simulink library "btb"  (Simulink 8.1)
settings: Solver=ode1  StartTime=0.0  StopTime=Inf  FixedStep=0.001  RelTol=1e-3
PostLoadFcn:
  | , if any(exist('dsrtsu_mdlpostloadfcn', 'file') == [2, 3, 6]), try dsrtsu_mdlpostloadfcn('Execute', bdroot); catch fprintf('Error in PostLoadFcn (dsrtsu_mdlpostloadfcn) for model "%s":\n %s\n', bdroot, lasterr); end, end,
undefined symbols (not defined in the file or in its folder): KACC_ACCDefBrakDist_m, KACC_ACCStopDistance_m, KACC_BrakeToStopConsideredDecel_mps2, KACC_BrakeToStopFreeRunTime_s
libraries: hcu_lib x2
settings Model: DSRTSU_INTERNAL_RTI_VER=450  DSRTSU_INTERNAL_RTI_TYPE=rti1401  Creator=AT015555  LastModifiedBy=AT015555

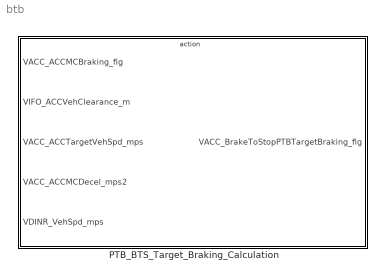
== system btb ==
  PTB_BTS_Target_Braking_Calculation : Subsystem  TreatAsAtomicUnit=on

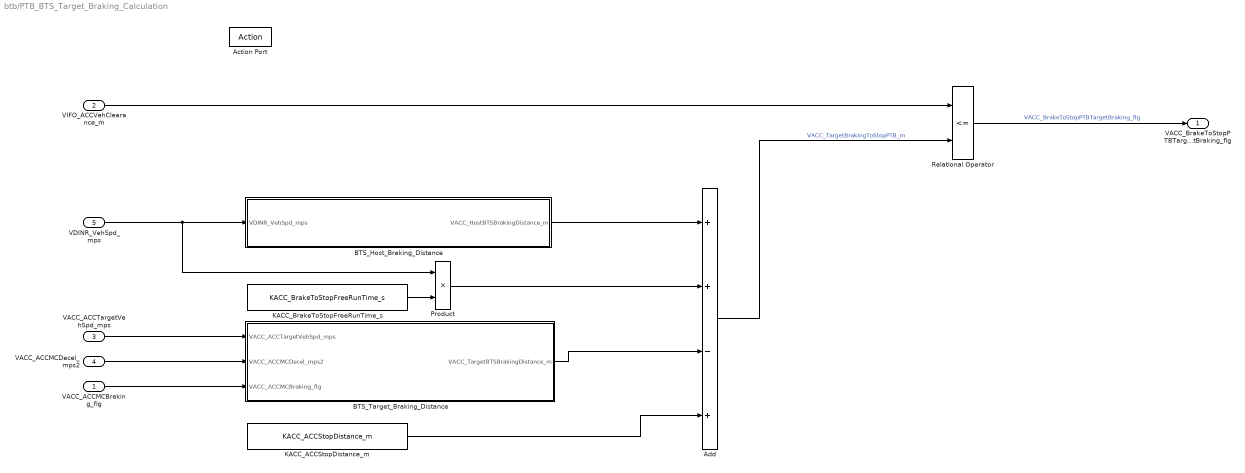
== system btb/PTB_BTS_Target_Braking_Calculation ==
  VACC_ACCMCBraking_flg : Inport
  VIFO_ACCVehClearance_m : Inport  Port=2
  VACC_ACCTargetVehSpd_mps : Inport  Port=3
  VACC_ACCMCDecel_mps2 : Inport  Port=4
  VDINR_VehSpd_mps : Inport  Port=5
  Action Port : ActionPort
  Add : Sum  Inputs=++-+
  BTS_Host_Braking_Distance : Subsystem
  BTS_Target_Braking_Distance : Subsystem
  KACC_ACCStopDistance_m : Constant  Value=KACC_ACCStopDistance_m
  KACC_BrakeToStopFreeRunTime_s : Constant  Value=KACC_BrakeToStopFreeRunTime_s
  Product : Product
  Relational Operator : RelationalOperator  Operator=<=  OutDataTypeStr=boolean
  VACC_BrakeToStopPTBTargetBraking_flg : Outport
  wires:
  VACC_ACCMCBraking_flg/1 -> BTS_Target_Braking_Distance/3(VACC_ACCMCBraking_flg)
  Relational Operator/1 -> VACC_BrakeToStopPTBTargetBraking_flg/1  "VACC_BrakeToStopPTBTargetBraking_flg"
  Add/1 -> Relational Operator/2  "VACC_TargetBrakingToStopPTB_m"
  VACC_ACCMCDecel_mps2/1 -> BTS_Target_Braking_Distance/2(VACC_ACCMCDecel_mps2)
  VACC_ACCTargetVehSpd_mps/1 -> BTS_Target_Braking_Distance/1(VACC_ACCTargetVehSpd_mps)
  BTS_Target_Braking_Distance/1(VACC_TargetBTSBrakingDistance_m) -> Add/3
  Product/1 -> Add/2
  KACC_BrakeToStopFreeRunTime_s/1 -> Product/2
  BTS_Host_Braking_Distance/1(VACC_HostBTSBrakingDistance_m) -> Add/1
  VDINR_VehSpd_mps/1 -> BTS_Host_Braking_Distance/1(VDINR_VehSpd_mps), Product/1
  KACC_ACCStopDistance_m/1 -> Add/4
  VIFO_ACCVehClearance_m/1 -> Relational Operator/1

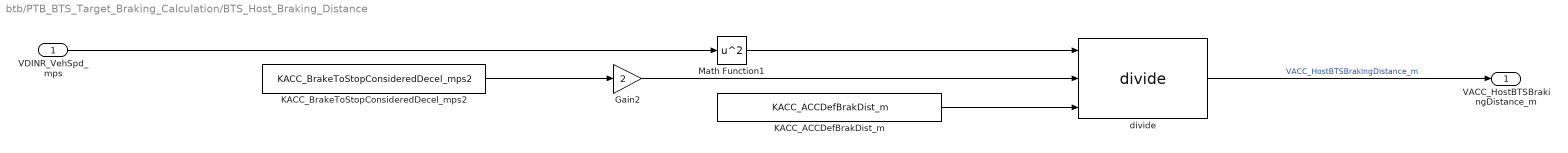
== system btb/PTB_BTS_Target_Braking_Calculation/BTS_Host_Braking_Distance ==
  VDINR_VehSpd_mps : Inport
  Gain2 : Gain  Gain=2
  KACC_ACCDefBrakDist_m : Constant  Value=KACC_ACCDefBrakDist_m
  KACC_BrakeToStopConsideredDecel_mps2 : Constant  Value=KACC_BrakeToStopConsideredDecel_mps2
  Math Function1 : Math  Operator=square  SaturateOnIntegerOverflow=on
  divide : hcu_lib/divide
  VACC_HostBTSBrakingDistance_m : Outport
  wires:
  KACC_BrakeToStopConsideredDecel_mps2/1 -> Gain2/1
  divide/1 -> VACC_HostBTSBrakingDistance_m/1  "VACC_HostBTSBrakingDistance_m"
  VDINR_VehSpd_mps/1 -> Math Function1/1
  KACC_ACCDefBrakDist_m/1 -> divide/3
  Gain2/1 -> divide/2
  Math Function1/1 -> divide/1

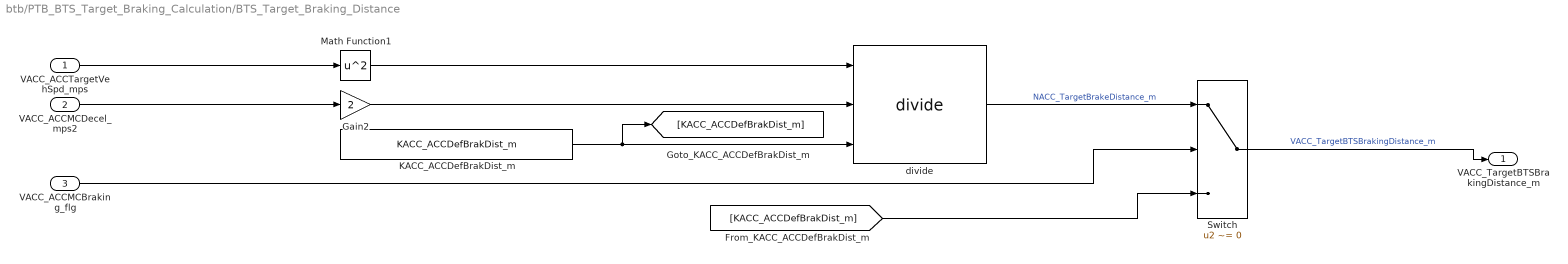
== system btb/PTB_BTS_Target_Braking_Calculation/BTS_Target_Braking_Distance ==
  VACC_ACCTargetVehSpd_mps : Inport
  VACC_ACCMCDecel_mps2 : Inport  Port=2
  VACC_ACCMCBraking_flg : Inport  Port=3
  Gain2 : Gain  Gain=2
  KACC_ACCDefBrakDist_m : Constant  Value=KACC_ACCDefBrakDist_m
  Math Function1 : Math  Operator=square  SaturateOnIntegerOverflow=on
  Switch : Switch  Criteria=u2 ~= 0
  divide : hcu_lib/divide
  VACC_TargetBTSBrakingDistance_m : Outport
  wires:
  [KACC_ACCDefBrakDist_m] -> Switch/3
  VACC_ACCMCBraking_flg/1 -> Switch/2
  divide/1 -> Switch/1  "NACC_TargetBrakeDistance_m"
  Math Function1/1 -> divide/1
  Gain2/1 -> divide/2
  KACC_ACCDefBrakDist_m/1 -> divide/3, [KACC_ACCDefBrakDist_m]
  VACC_ACCTargetVehSpd_mps/1 -> Math Function1/1
  Switch/1 -> VACC_TargetBTSBrakingDistance_m/1  "VACC_TargetBTSBrakingDistance_m"
  VACC_ACCMCDecel_mps2/1 -> Gain2/1
